simulink model "unicycles_clean"  (R2018b)
settings: Solver=FixedStepAuto  StartTime=0.0  StopTime=20  FixedStep=1e-3  RelTol=1e-3  EnableMultiTasking=on
InitFcn:
  | init_unicycle_car_ineq
values from neighbouring files (symbols this model uses):
  dmax = 2    [init_unicycle_car_ineq.m]
  dmin = 1    [init_unicycle_car_ineq.m]
  th1 = pi/4    (= 0.785398163397)    [init_unicycle_car_ineq.m]
  th2 = pi/4    (= 0.785398163397)    [init_unicycle_car_ineq.m]
  th3 = 3*pi/4    (= 2.35619449019)    [init_unicycle_car_ineq.m]
  x1 = 2    [init_unicycle_car_ineq.m]
  x2 = 0.9    [init_unicycle_car_ineq.m]
  x3 = 3.1    [init_unicycle_car_ineq.m]
  y1 = 2    [init_unicycle_car_ineq.m]
  y2 = 0.9    [init_unicycle_car_ineq.m]
  y3 = 0.9    [init_unicycle_car_ineq.m]
settings Model: Creator=Jim  LastModifiedBy=ahmed
settings DataIOCC: LimitDataPoints=on  SaveFormat=Array
settings OptimizationCC: LifeSpan=inf
settings DebuggingCC: SFUnexpectedBacktrackingDiag=warning  SFNoUnconditionalDefaultTransitionDiag=warning  SFExecutionAtInitializationDiag=none
settings HardwareCC: ProdBitPerPointer=32  ProdBitPerSizeT=32  ProdBitPerPtrDiffT=32  ProdLargestAtomicFloat=None  ProdIntDivRoundTo=Undefined  ProdEndianess=Unspecified  ProdWordSize=32  ProdHWDeviceType=32-bit Generic
settings ModelReferenceCC: PropagateSignalLabelsOutOfModel=off
settings SFSimCC: SimUseLocalCustomCode=off
settings RTWCC: RTWUseLocalCustomCode=off
settings CodeAppCC: StateflowObjectComments=on
settings GRTTargetCC: TargetLangStandard=C89/C90 (ANSI)  GeneratePreprocessorConditionals=Disable all
settings ConfigComp: CovMetricSettings=dw  CovHtmlReporting=on  CovSaveCumulativeToWorkspaceVar=on  CovSaveSingleToWorkspaceVar=on  CovExternalEMLEnable=off

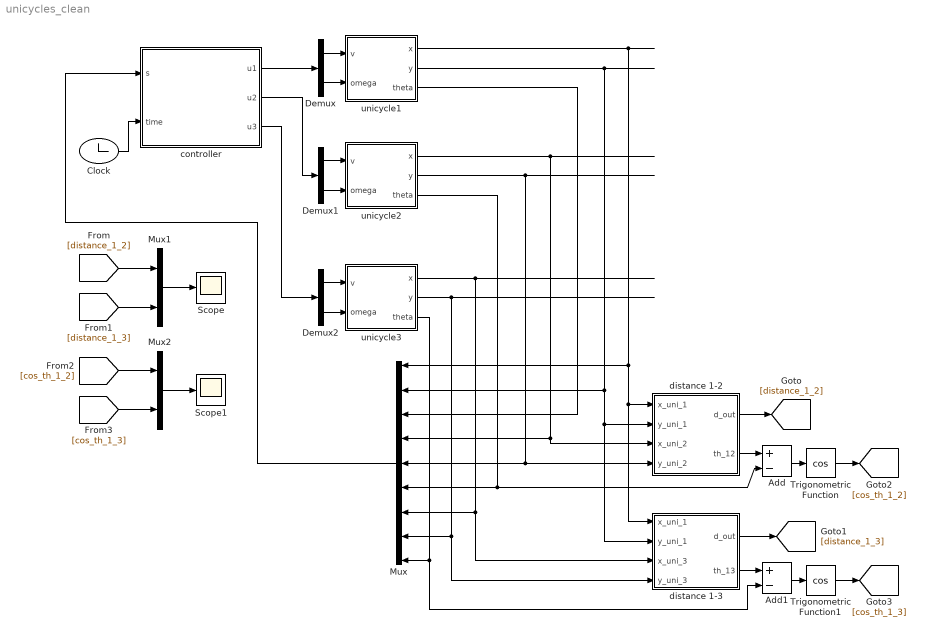
== system unicycles_clean ==
  Add : Sum  Inputs=+-
  Add1 : Sum  Inputs=+-
  Clock : Clock
  Demux : Demux  Outputs=2
  Demux1 : Demux  Outputs=2
  Demux2 : Demux  Outputs=2
  Mux : Mux  Inputs=9
  Mux1 : Mux  Inputs=2
  Mux2 : Mux  Inputs=2
  Scope : Scope
  Scope1 : Scope
  Trigonometric Function : Trigonometry  Operator=cos
  Trigonometric Function1 : Trigonometry  Operator=cos
  controller : MATLAB Function  TreatAsAtomicUnit=on
  distance 1-2 : Subsystem
  distance 1-3 : Subsystem
  unicycle1 : Subsystem
  unicycle2 : Subsystem
  unicycle3 : Subsystem
  wires:
  unicycle1/1(x) -> distance 1-3/1(x_uni_1), distance 1-2/1(x_uni_1), Mux/1
  unicycle1/2(y) -> distance 1-3/2(y_uni_1), distance 1-2/2(y_uni_1), Mux/2
  unicycle1/3(theta) -> Mux/3
  controller/1(u1) -> Demux/1
  Demux/1 -> unicycle1/1(v)
  Demux/2 -> unicycle1/2(omega)
  Demux1/1 -> unicycle2/1(v)
  Demux1/2 -> unicycle2/2(omega)
  Demux2/1 -> unicycle3/1(v)
  Demux2/2 -> unicycle3/2(omega)
  controller/2(u2) -> Demux1/1
  controller/3(u3) -> Demux2/1
  unicycle2/1(x) -> distance 1-2/3(x_uni_2), Mux/4
  unicycle2/2(y) -> distance 1-2/4(y_uni_2), Mux/5
  unicycle3/1(x) -> distance 1-3/3(x_uni_3), Mux/7
  unicycle3/2(y) -> Mux/8, distance 1-3/4(y_uni_3)
  Mux/1 -> controller/1(s)
  Clock/1 -> controller/2(time)
  distance 1-2/2(th_12) -> Add/1
  distance 1-3/2(th_13) -> Add1/1
  unicycle2/3(theta) -> Add/2, Mux/6
  unicycle3/3(theta) -> Add1/2, Mux/9
  Add/1 -> Trigonometric Function/1
  Add1/1 -> Trigonometric Function1/1
  Mux1/1 -> Scope/1
  Mux2/1 -> Scope1/1
  distance 1-2/1(d_out) -> [distance_1_2]
  [distance_1_2] -> Mux1/1
  distance 1-3/1(d_out) -> [distance_1_3]
  Trigonometric Function/1 -> [cos_th_1_2]
  Trigonometric Function1/1 -> [cos_th_1_3]
  [distance_1_3] -> Mux1/2
  [cos_th_1_3] -> Mux2/2
  [cos_th_1_2] -> Mux2/1

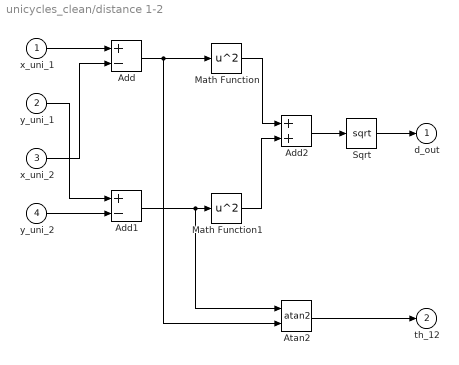
== system unicycles_clean/distance 1-2 ==
  x_uni_1 : Inport
  y_uni_1 : Inport  Port=2
  x_uni_2 : Inport  Port=3
  y_uni_2 : Inport  Port=4
  Add : Sum  Inputs=+-
  Add1 : Sum  Inputs=+-
  Add2 : Sum
  Atan2 : Trigonometry  Operator=atan2
  Math Function : Math  Operator=square  SaturateOnIntegerOverflow=on
  Math Function1 : Math  Operator=square  SaturateOnIntegerOverflow=on
  Sqrt : Sqrt  SaturateOnIntegerOverflow=on
  d_out : Outport
  th_12 : Outport  Port=2
  wires:
  x_uni_1/1 -> Add/1
  x_uni_2/1 -> Add/2
  y_uni_2/1 -> Add1/2
  y_uni_1/1 -> Add1/1
  Add/1 -> Math Function/1, Atan2/2
  Add1/1 -> Atan2/1, Math Function1/1
  Math Function/1 -> Add2/1
  Math Function1/1 -> Add2/2
  Add2/1 -> Sqrt/1
  Sqrt/1 -> d_out/1
  Atan2/1 -> th_12/1

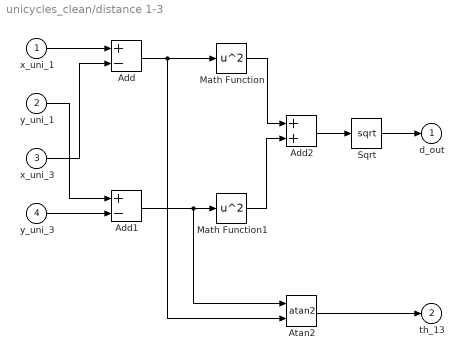
== system unicycles_clean/distance 1-3 ==
  x_uni_1 : Inport
  y_uni_1 : Inport  Port=2
  x_uni_3 : Inport  Port=3
  y_uni_3 : Inport  Port=4
  Add : Sum  Inputs=+-
  Add1 : Sum  Inputs=+-
  Add2 : Sum
  Atan2 : Trigonometry  Operator=atan2
  Math Function : Math  Operator=square  SaturateOnIntegerOverflow=on
  Math Function1 : Math  Operator=square  SaturateOnIntegerOverflow=on
  Sqrt : Sqrt  SaturateOnIntegerOverflow=on
  d_out : Outport
  th_13 : Outport  Port=2
  wires:
  x_uni_1/1 -> Add/1
  x_uni_3/1 -> Add/2
  y_uni_3/1 -> Add1/2
  y_uni_1/1 -> Add1/1
  Add/1 -> Atan2/2, Math Function/1
  Add1/1 -> Atan2/1, Math Function1/1
  Math Function/1 -> Add2/1
  Math Function1/1 -> Add2/2
  Add2/1 -> Sqrt/1
  Sqrt/1 -> d_out/1
  Atan2/1 -> th_13/1

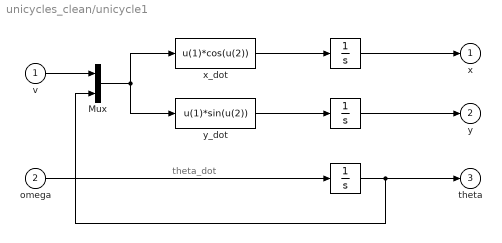
== system unicycles_clean/unicycle1 ==
  note: theta_dot
  v : Inport
  omega : Inport  Port=2
  " " : Integrator  InitialCondition=th1
  "   " : Integrator  InitialCondition=x1
  "    " : Integrator  InitialCondition=y1
  Mux : Mux  Inputs=2
  x_dot : Fcn  Expr=u(1)*cos(u(2))
  y_dot : Fcn  Expr=u(1)*sin(u(2))
  x : Outport
  y : Outport  Port=2
  theta : Outport  Port=3
  wires:
  v/1 -> Mux/1
  omega/1 -> " "/1
  x_dot/1 -> "   "/1
  y_dot/1 -> "    "/1
  " "/1 -> Mux/2, theta/1
  Mux/1 -> x_dot/1, y_dot/1
  "   "/1 -> x/1
  "    "/1 -> y/1

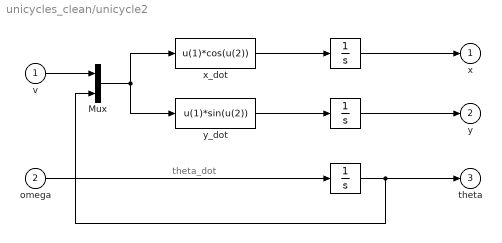
== system unicycles_clean/unicycle2 ==
  note: theta_dot
  v : Inport
  omega : Inport  Port=2
  " " : Integrator  InitialCondition=th2
  "   " : Integrator  InitialCondition=x2
  "    " : Integrator  InitialCondition=y2
  Mux : Mux  Inputs=2
  x_dot : Fcn  Expr=u(1)*cos(u(2))
  y_dot : Fcn  Expr=u(1)*sin(u(2))
  x : Outport
  y : Outport  Port=2
  theta : Outport  Port=3
  wires:
  v/1 -> Mux/1
  omega/1 -> " "/1
  x_dot/1 -> "   "/1
  y_dot/1 -> "    "/1
  " "/1 -> Mux/2, theta/1
  Mux/1 -> x_dot/1, y_dot/1
  "   "/1 -> x/1
  "    "/1 -> y/1

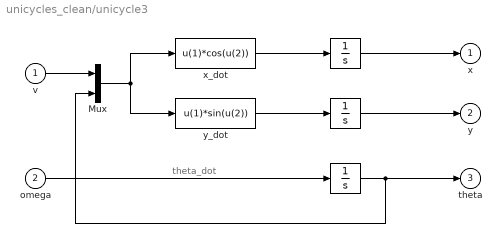
== system unicycles_clean/unicycle3 ==
  note: theta_dot
  v : Inport
  omega : Inport  Port=2
  " " : Integrator  InitialCondition=th3
  "   " : Integrator  InitialCondition=x3
  "    " : Integrator  InitialCondition=y3
  Mux : Mux  Inputs=2
  x_dot : Fcn  Expr=u(1)*cos(u(2))
  y_dot : Fcn  Expr=u(1)*sin(u(2))
  x : Outport
  y : Outport  Port=2
  theta : Outport  Port=3
  wires:
  v/1 -> Mux/1
  omega/1 -> " "/1
  x_dot/1 -> "   "/1
  y_dot/1 -> "    "/1
  " "/1 -> Mux/2, theta/1
  Mux/1 -> x_dot/1, y_dot/1
  "   "/1 -> x/1
  "    "/1 -> y/1

== matlab function unicycles_clean/controller ==
  settings: updateMethod=DISCRETE
  data: s input size=9; time input; u1 output size=2; u2 output size=2; u3 output; dmin parameter; dmax parameter
function [u1, u2, u3] = fcn(s, time, dmin, dmax)

%unpacking state vector
x1 = s(1);
y1 = s(2);
th1 = s(3);
x2 = s(4);
y2 = s(5);
th2 = s(6);
x3 = s(7);
y3 = s(8);
th3 = s(9);

v1r = 2*sin(time);
u1r = 2*cos(2*time);
% v1r = sin(time);
% u1r = cos(2*time);
alpha12 = 0.4;
alpha13 = 0.4;
u1 = [v1r; u1r];
u2 = [0; 0];
u3 = [0; 0];

K_bar = [cos(th1)*v1r; sin(th1)*v1r; u1r; 0; 0; 0; 0; 0; 0];
K1 = [0; 0; 0; 0;        0;        1; 0;        0;        0];
K2 = [0; 0; 0; 0;        0;        0; 0;        0;        1];
K3 = [0; 0; 0; cos(th2); sin(th2); 0; 0;        0;        0];
K4 = [0; 0; 0; 0;        0;        0; cos(th3); sin(th3); 0];
K = [K1 K2 K3 K4];

% w1 = omega2; w2 = omega3; w3 = v2; w4 = v3;
a = -1; b = 1;
w = a + (b-a).*rand(1,4);

vel = -8:1:8;

% Check active constraints
I12_1_r = (x1-x2)^2+(y1-y2)^2 - dmax^2;
I12_1_l = dmin^2 - ((x1-x2)^2+(y1-y2)^2);
d12 = sqrt((x1-x2)^2+(y1-y2)^2);
I12_2 = cos(alpha12)*d12 - ((x1-x2)*cos(th2)+(y1-y2)*sin(th2));

I13_1_r = (x1-x3)^2+(y1-y3)^2 - dmax^2;
I13_1_l = dmin^2 - ((x1-x3)^2+(y1-y3)^2);
d13 = sqrt((x1-x3)^2+(y1-y3)^2);
I13_2 = cos(alpha13)*d13 - ((x1-x3)*cos(th3)+(y1-y3)*sin(th3));

I23 = 0.25^2 - ((x3-x2)^2+(y3-y2)^2);

I12 = [I12_1_r I12_1_l I12_2 I23];
I13 = [I13_1_r I13_1_l I13_2];

% w1 = omega2; w2 = omega3; w3 = v2; w4 = v3;
if sum(I12(:)>=0)==0
    u2 = [w(3);  w(1)];
else
    n = 0;
    while true
        pd = K_bar + K(:,1)*w(1) + K(:,3)*w(3);
        x1d = pd(1); y1d = pd(2); th1d = pd(3);
        x2d = pd(4); y2d = pd(5); th2d = pd(6);
        x3d = pd(7); y3d = pd(8); th3d = pd(9);
        
        sigma_I_12_1_r = (x1-x2)*(x1d-x2d)+(y1-y2)*(y1d-y2d);
        sigma_I_12_1_l = -((x1-x2)*(x1d-x2d)+(y1-y2)*(y1d-y2d));
        sigma_I_12_2 = (cos(alpha12)*((x1-x2)*(x1d-x2d)+(y1-y2)*(y1d-y2d))/d12)-...
            (x1d-x2d)*cos(th2)-(y1d-y2d)*sin(th2)+...
            (x1-x2)*sin(th2)*th2d-(y1-y2)*cos(th2)*th2d;
        sigma_I_23 = -((x3-x2)*(x3d-x2d)+(y3-y2)*(y3d-y2d));
        
        sigma_I = [sigma_I_12_1_r sigma_I_12_1_l sigma_I_12_2 sigma_I_23];
        
        u2 = [0; 0];
        if all(sigma_I(I12>=0) <= 0)
            u2 = [w(3);  w(1)];
            break;
        end
        
        w(3) = vel(randi([1, length(vel)]));
        w(1) = vel(randi([1, length(vel)]));
        if n>100
            z=time;
        end
        n = n+1;
    end
end

% w1 = omega2; w2 = omega3; w3 = v2; w4 = v3;
if sum(I13(:)>=0)==0
    u3 = [w(4);  w(2)];
else
    n = 0;
    while true
        pd = K_bar + K(:,2)*w(2) + K(:,4)*w(4);
        x1d = pd(1); y1d = pd(2); th1d = pd(3);
        x2d = pd(4); y2d = pd(5); th2d = pd(6);
        x3d = pd(7); y3d = pd(8); th3d = pd(9);
        
        sigma_I_13_1_r = (x1-x3)*(x1d-x3d)+(y1-y3)*(y1d-y3d);
        sigma_I_13_1_l = -((x1-x3)*(x1d-x3d)+(y1-y3)*(y1d-y3d));
        sigma_I_13_2 = (cos(alpha13)*((x1-x3)*(x1d-x3d)+(y1-y3)*(y1d-y3d))/d13)-...
            (x1d-x3d)*cos(th3)-(y1d-y3d)*sin(th3)+...
            (x1-x3)*sin(th3)*th3d-(y1-y3)*cos(th3)*th3d;
        
        sigma_I = [sigma_I_13_1_r sigma_I_13_1_l sigma_I_13_2];
        
        u3 = [0; 0];
        if all(sigma_I(I13>=0) <= 0)
            u3 = [w(4);  w(2)];
            break;
        end
        
        w(4) = vel(randi([1, length(vel)]));
        w(2) = vel(randi([1, length(vel)]));        
        if n>100
            z=time;
        end
        n = n+1;
    end
end
